simulink model "Qmoddef"
settings: Solver=ode45  StartTime=0.0  StopTime=10.0  RelTol=1e-3
undefined symbols (not defined in the file or in its folder): Ax, Ay, Az, g, Ixx, Iyy, Izz, k, l, m
settings Model: Creator=DNI 38876767  LastModifiedBy=gabriel
settings DataIOCC: LimitDataPoints=on  SaveFormat=Array  ReturnWorkspaceOutputs=off
settings OptimizationCC: ExpressionDepthLimit=2147483647  LifeSpan=inf  SimCompilerOptimization=Off
settings DebuggingCC: UnderspecifiedInitializationDetection=Classic  MergeDetectMultiDrivingBlocksExec=none  SolverPrmCheckMsg=warning  MultiTaskDSMMsg=warning  MultiTaskCondExecSysMsg=none  FcnCallInpInsideContextMsg=Enable All  FrameProcessingCompatibilityMsg=warning  StateNameClashWarn=warning  StrictBusMsg=None  SFUnexpectedBacktrackingDiag=warning  SFNoUnconditionalDefaultTransitionDiag=warning
settings HardwareCC: ProdBitPerPointer=32  ProdLargestAtomicFloat=None  ProdIntDivRoundTo=Undefined  ProdEndianess=Unspecified  ProdWordSize=32  ProdHWDeviceType=32-bit Generic
settings ModelReferenceCC: PropagateSignalLabelsOutOfModel=off
settings SFSimCC: SimUseLocalCustomCode=off
settings RTWCC: RTWUseLocalCustomCode=off  IncludeERTFirstTime=on  RTWCompilerOptimization=Off
settings CodeAppCC: CustomSymbolStrType=$N$R$M
settings GRTTargetCC: CodeReplacementLibrary=ANSI_C  GeneratePreprocessorConditionals=Disable all  CPPClassGenCompliant=off

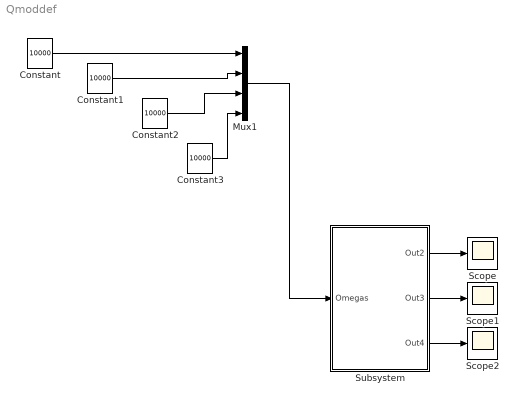
== system Qmoddef ==
  Constant{,1..3} (4 alike) : Constant  Value=10000
  Mux1 : Mux
  Scope : Scope
  Scope1 : Scope
  Scope2 : Scope
      settings: SaveName=ScopeData2
  Subsystem : Subsystem
  wires:
  Mux1/1 -> Subsystem/1("Omegas ")
  Subsystem/1(Out2) -> Scope/1
  Subsystem/2(Out3) -> Scope1/1
  Subsystem/3(Out4) -> Scope2/1
  Constant/1 -> Mux1/1
  Constant1/1 -> Mux1/2
  Constant2/1 -> Mux1/3
  Constant3/1 -> Mux1/4

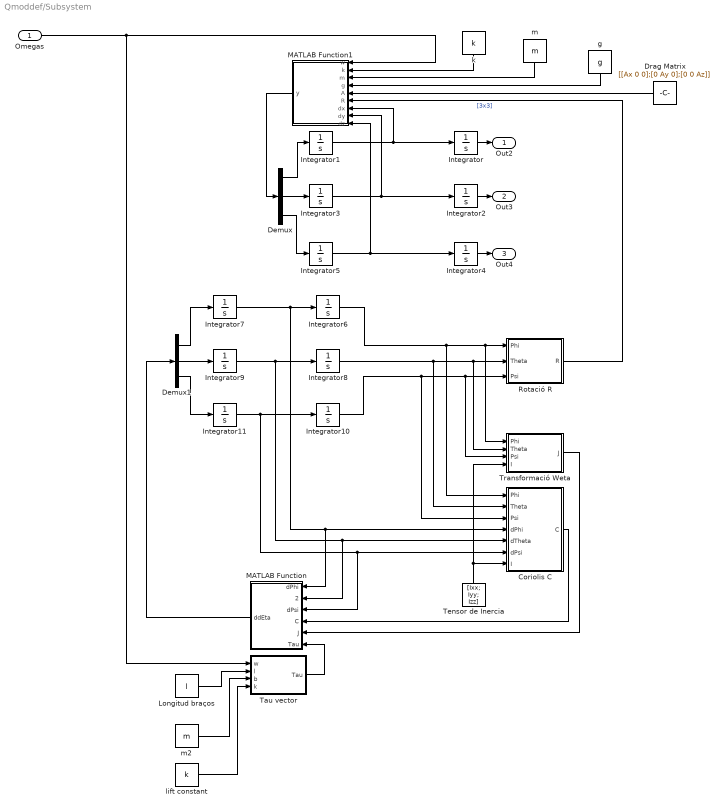
== system Qmoddef/Subsystem ==
  "Omegas " : Inport
  Coriolis C : MATLAB Function  TreatAsAtomicUnit=on
  Demux : Demux  Outputs=3
  Demux1 : Demux  Outputs=3
  Drag Matrix : Constant  Value=[[Ax 0 0];[0 Ay 0];[0 0 Az]]
  Integrator{,2..11} (11 alike) : Integrator
  Integrator1 : Integrator  InitialCondition=1
  Longitud braços : Constant  Value=l
  MATLAB Function : MATLAB Function  TreatAsAtomicUnit=on
  MATLAB Function1 : MATLAB Function  TreatAsAtomicUnit=on
  Rotació R : MATLAB Function  TreatAsAtomicUnit=on
  Tau vector : MATLAB Function  TreatAsAtomicUnit=on
  Tensor de Inercia : Constant  Value=[Ixx; Iyy; Izz]
  "Transformació Weta " : MATLAB Function  TreatAsAtomicUnit=on
  "g " : Constant  Value=g
  k : Constant  Value=k
  lift constant : Constant  Value=k
  m : Constant  Value=m
  m2 : Constant  Value=m
  Out2 : Outport
  Out3 : Outport  Port=2
  Out4 : Outport  Port=3
  wires:
  Integrator9/1 -> MATLAB Function/2(dTheta), Coriolis C/5(dTheta), Integrator8/1
  MATLAB Function1/1(y) -> Demux/1
  Integrator11/1 -> MATLAB Function/3(dPsi), Coriolis C/6(dPsi), Integrator10/1
  Integrator5/1 -> Integrator4/1, MATLAB Function1/9(dz)
  Integrator7/1 -> MATLAB Function/1(dPhi), Coriolis C/4(dPhi), Integrator6/1
  Integrator3/1 -> Integrator2/1, MATLAB Function1/8(dy)
  Integrator/1 -> Out2/1
  Demux1/1 -> Integrator7/1
  Rotació R/1(R) -> MATLAB Function1/6(R)  "[3x3]"
  Integrator4/1 -> Out4/1
  Demux1/3 -> Integrator11/1
  Integrator2/1 -> Out3/1
  Demux1/2 -> Integrator9/1
  "Omegas "/1 -> Tau vector/1(w), MATLAB Function1/1(w)
  Demux/3 -> Integrator5/1
  Integrator8/1 -> Coriolis C/2(Theta), "Transformació Weta "/2(Theta), Rotació R/2(Theta)
  Demux/1 -> Integrator1/1
  Demux/2 -> Integrator3/1
  Integrator1/1 -> Integrator/1, MATLAB Function1/7(dx)
  Integrator10/1 -> Coriolis C/3(Psi), "Transformació Weta "/3(Psi), Rotació R/3(Psi)
  Integrator6/1 -> Coriolis C/1(Phi), "Transformació Weta "/1(Phi), Rotació R/1(Phi)
  k/1 -> MATLAB Function1/2(k)
  Tensor de Inercia/1 -> "Transformació Weta "/4(I), Coriolis C/7(I)
  m/1 -> MATLAB Function1/3(m)
  "g "/1 -> MATLAB Function1/4(g)
  Coriolis C/1(C) -> MATLAB Function/4(C)
  Longitud braços/1 -> Tau vector/2(l)
  m2/1 -> Tau vector/3(b)
  lift constant/1 -> Tau vector/4(k)
  Tau vector/1(Tau) -> MATLAB Function/6(Tau)
  "Transformació Weta "/1(J) -> MATLAB Function/5(J)
  MATLAB Function/1(ddEta) -> Demux1/1
  Drag Matrix/1 -> MATLAB Function1/5(A)

== matlab function Qmoddef/Subsystem/MATLAB Function1 ==
  data: w input; k input; m input; g input; A input; y output; R input; dx input; dy input; dz input
function y = fcn(w,k,m,g,A,R,dx,dy,dz)
%#codegen

Thrust=[0; 0; k*(w(1)*w(1)+w(2)*w(2)+w(3)*w(3)+w(4)*w(4))/m];


y=R*Thrust-[0; 0; g]-A*[dx; dy; dz]/m;

== matlab function Qmoddef/Subsystem/Rotació R ==
  data: Phi input; R output; Theta input; Psi input
function R = fcn(Phi,Theta,Psi)
%#codegen
%H=sym('H')
R = [[cos(Psi)*cos(Theta) cos(Psi)*sin(Theta)*sin(Phi)-sin(Psi)*cos(Phi) cos(Psi)*sin(Theta)*cos(Phi)+sin(Psi)*sin(Phi)];
     [sin(Psi)*cos(Theta) sin(Psi)*sin(Theta)*sin(Phi)+cos(Psi)*cos(Phi) sin(Psi)*sin(Theta)*cos(Phi)-cos(Psi)*sin(Phi)];
     [-sin(Theta) cos(Theta)*sin(Phi) cos(Theta)*cos(Phi)]];

== matlab function Qmoddef/Subsystem/Coriolis C ==
  data: Phi input; Theta input; Psi input; C output; dPhi input; dTheta input; dPsi input; I input
function C = fcn(Phi,Theta,Psi,dPhi,dTheta,dPsi,I)
%#codegen

Ixx=I(1);
Iyy=I(2);
Izz=I(3);

C11=0;
C12=(Iyy-Izz)*(dTheta*cos(Phi)*sin(Phi)+dPsi*sin(Phi)*sin(Phi)*cos(Theta))+(Izz-Iyy)*dPsi*cos(Phi)*cos(Phi)*cos(Theta)-Ixx*dPsi*cos(Theta);
C13=(Izz-Iyy)*dPsi*cos(Phi)*sin(Phi)*(cos(Theta)^2);

% C21=(Izz-Iyy)*(dTheta*cos(Phi)*sin(Phi)+dPsi*(sin(Phi)^2)*cos(Theta))+(Izz-Iyy)*dPsi*(cos(Phi)^2)*cos(Theta)-Ixx*dPsi*cos(Theta);
C21=(Izz-Iyy)*(dTheta*cos(Phi)*sin(Phi)+dPsi*sin(Phi)*cos(Theta))+(Iyy-Izz)*dPsi*cos(Phi)*cos(Phi)*cos(Theta)+Ixx*dPsi*cos(Theta);
C22=(Izz-Iyy)*dPhi*cos(Phi)*sin(Phi);
C23=-Ixx*dPsi*sin(Theta)*cos(Theta)+Iyy*dPsi*sin(Phi)*sin(Phi)*sin(Theta)*cos(Theta)+Izz*dPsi*cos(Phi)*cos(Phi)*sin(Theta)*cos(Theta);

C31=(Iyy-Izz)*dPsi*cos(Theta)*cos(Theta)*sin(Phi)*cos(Phi)-Ixx*dTheta*cos(Theta);
C32=(Izz-Iyy)*(dTheta*cos(Phi)*sin(Phi)*sin(Theta)+dPhi*sin(Phi)*sin(Phi)*cos(Theta))+(Iyy-Izz)*dPhi*cos(Phi)*cos(Phi)*cos(Theta)+Ixx*dPsi*sin(Theta)*cos(Theta)-Iyy*dPsi*sin(Phi)*sin(Phi)*sin(Theta)*cos(Theta)-Izz*dPsi*cos(Phi)*cos(Phi)*sin(Theta)*cos(Theta);
C33=(Iyy-Izz)*dPhi*cos(Phi)*sin(Phi)*cos(Theta)*cos(Theta)-Iyy*dTheta*sin(Phi)*sin(Phi)*cos(Theta)*sin(Theta)-Izz*dTheta*cos(Phi)*cos(Phi)*cos(Theta)*sin(Theta)+Ixx*dTheta*cos(Theta)*sin(Theta);

Cmat=[[C11 C12 C13];
   [C21 C22 C23];
   [C31 C32 C33]];

C = Cmat;

== matlab function Qmoddef/Subsystem/Transformació Weta  ==
  data: Phi input; Theta input; Psi input; J output; I input
function J = fcn(Phi,Theta,Psi,I)
%#codegen

Ixx=I(1);
Iyy=I(2);
Izz=I(3);

Weta=[[1 0 -sin(Theta)];
      [0 cos(Phi) cos(Theta)*sin(Phi)];
      [0 -sin(Phi) cos(Theta)*cos(Phi)]];
  
WetaT=transpose(Weta);

II=[[Ixx 0 0];[0 Iyy 0];[0 0 Izz]];

J = WetaT*II*Weta;

== matlab function Qmoddef/Subsystem/MATLAB Function ==
  data: dPhi input; dTheta input; dPsi input; ddEta output; C input; J input; Tau input
function ddEta = fcn(dPhi,dTheta,dPsi,C,J,Tau)
%#codegen

ddEta = inv(J)*(Tau-C*[dPhi; dTheta; dPsi]);

== matlab function Qmoddef/Subsystem/Tau vector ==
  data: w input; Tau output; l input; b input; k input
function Tau = fcn(w,l,b,k)
%#codegen

Tau = [l*k*(w(4)^2-w(2)^2);
     l*k*(w(3)^2 - w(1)^2);
     b*(w(1)^2-w(2)^2+w(3)^2-w(4)^2)];
